simulink model "Number5"  (R2023b)
settings: Solver=VariableStepAuto  StartTime=0.0  StopTime=20.0  RelTol=1e-3
values from neighbouring files (symbols this model uses):
  G_den5 = [1 2 3 4 5 6 7 1]    [Malabanan_Problem5and6.m]
  G_num5 = [8 7 6 5 4 3 2]    [Malabanan_Problem5and6.m]
settings Model: Creator=angel  LastModifiedBy=angel

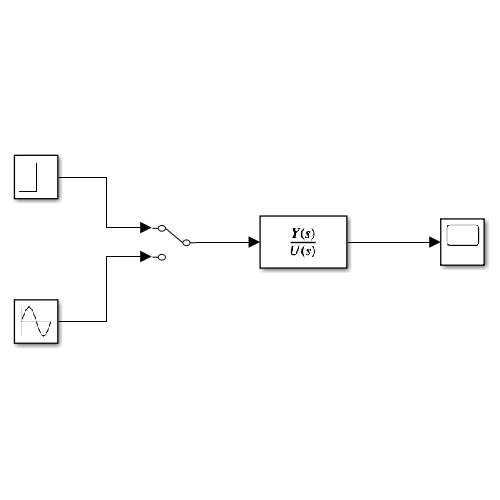
[thumbnail: Simulink's stored preview of the top-level diagram]
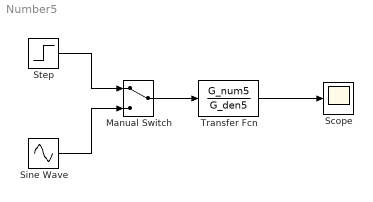
== system Number5 ==
  Manual Switch : ManualSwitch
  Scope : Scope
  Sine Wave : Sin  Frequency=20  SampleTime=0
  Step : Step  Time=0  SampleTime=0
  Transfer Fcn : TransferFcn  Numerator=G_num5  Denominator=G_den5
  wires:
  Transfer Fcn/1 -> Scope/1
  Step/1 -> Manual Switch/1
  Sine Wave/1 -> Manual Switch/2
  Manual Switch/1 -> Transfer Fcn/1
